simulink model "PID1"  (R2023b)
settings: Solver=VariableStepAuto  StartTime=0.0  StopTime=100  RelTol=1e-3
settings Model: Creator=86189  LastModifiedBy=86189

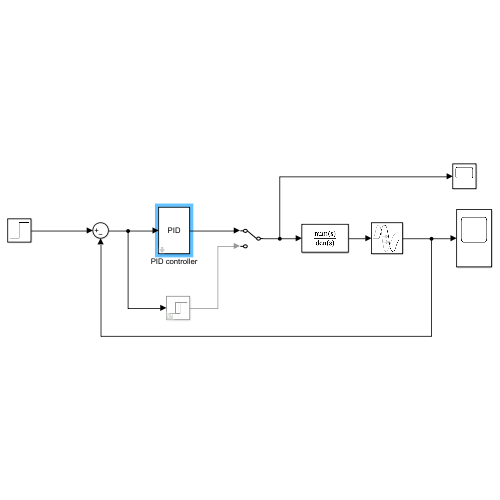
[thumbnail: Simulink's stored preview of the top-level diagram]
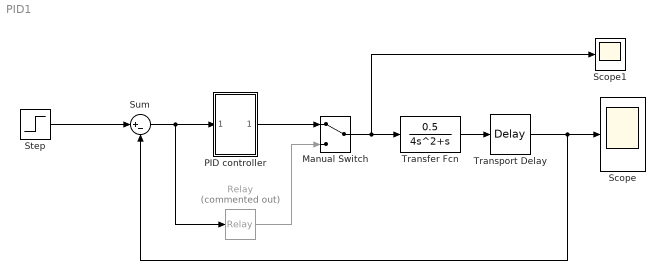
== system PID1 ==
  Manual Switch : ManualSwitch
  PID controller : Subsystem  mask{K_c=0.38, T_u=32}
      mask DialogControl ParameterGroupVar Prompt: 参数
      mask Display: disp('PID')
  Relay : Relay  Commented=on  OnSwitchValue=1  OffSwitchValue=-1  OnOutputValue=2  OffOutputValue=-2
  Scope : Scope
  Scope1 : Scope
  Step : Step  Time=10  SampleTime=0
  Sum : Sum  Inputs=|+-
  Transfer Fcn : TransferFcn  Numerator=[0.5]  Denominator=[4 1 0]
  Transport Delay : TransportDelay  DelayTime=2
  wires:
  Sum/1 -> Relay/1, PID controller/1(In1)
  PID controller/1(Out1) -> Manual Switch/1
  Transport Delay/1 -> Sum/2, Scope/1
  Relay/1 -> Manual Switch/2
  Manual Switch/1 -> Scope1/1, Transfer Fcn/1
  Transfer Fcn/1 -> Transport Delay/1
  Step/1 -> Sum/1

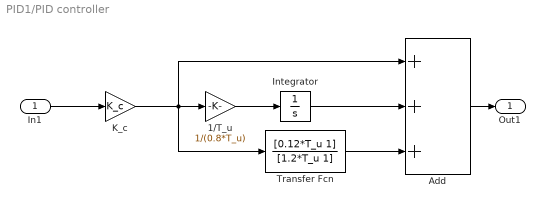
== system PID1/PID controller ==
  In1 : Inport
  1/T_u : Gain  Gain=1/(0.8*T_u)
  Add : Sum  Inputs=+++
  Integrator : Integrator
  K_c : Gain  Gain=K_c
  Transfer Fcn : TransferFcn  Numerator=[0.12*T_u 1]  Denominator=[1.2*T_u 1]
  Out1 : Outport
  wires:
  K_c/1 -> Add/1, Transfer Fcn/1, 1/T_u/1
  1/T_u/1 -> Integrator/1
  Add/1 -> Out1/1
  In1/1 -> K_c/1
  Integrator/1 -> Add/2
  Transfer Fcn/1 -> Add/3
